simulink model "spacecraft_animation"  (Simulink 9.2)
settings: Solver=ode45  StartTime=0.0  StopTime=10000  RelTol=1e-3  EnableMultiTasking=on
undefined symbols (not defined in the file or in its folder): drawSpacecraft
libraries: simulink x6
settings Model: Creator=beard  LastModifiedBy=beard
settings OptimizationCC: ExpressionDepthLimit=2147483647  InitFltsAndDblsToZero=on
settings DebuggingCC: SolverPrmCheckMsg=warning
settings GRTTargetCC: GeneratePreprocessorConditionals=Use local settings
settings ConfigComp: CovExternalEMLEnable=on

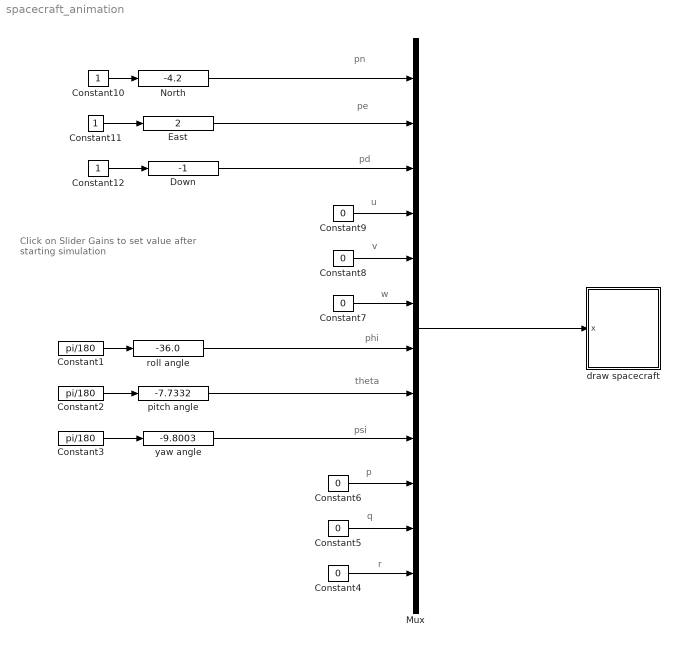
== system spacecraft_animation ==
  note: pn
  note: pe
  note: pd
  note: phi
  note: theta
  note: psi
  note: p
  note: q
  note: r
  note: u
  note: v
  note: w
  note: Click on Slider Gains to set value
      | after starting simulation
  Constant1 : Constant  Value=pi/180
  Constant10 : Constant
  Constant11 : Constant
  Constant12 : Constant
  Constant2 : Constant  Value=pi/180
  Constant3 : Constant  Value=pi/180
  Constant{4..9} (6 alike) : Constant  Value=0
  Down : simulink/Math Operations/Slider Gain  gain=-1  low=-10  high=10
  East : simulink/Math Operations/Slider Gain  gain=2  low=-10  high=10
  Mux : Mux  Inputs=12
  North : simulink/Math Operations/Slider Gain  gain=-4.2  low=-10  high=10
  draw spacecraft : Subsystem
      mask init:
      | % Define the vertices (physical location of vertices
      |   V = [...
      | 	 1    1    0;... % point 1
      |      1   -1    0;... % point 2
      |     -1   -1    0;... % point 3
      |     -1    1    0;... % point 4
      | 	 1    1   -2;... % point 5
      |      1   -1   -2;... % point 6
      |     -1   -1   -2;... % point 7
      |     -1    1   -2;... % point 8
      | 	 1.5  1.5  0;... % point 9
      |      1.5 -1.5  0;... % point 10
      |     -1.5 -1.5  0;... % point 11
      |     -1.5  1.5  0;... % point 12
      |   ];
      | 
      | % define faces as a list of vertices numbered above
      |   F = [...
      |         1, 2,  6,  5;...  % front
      |         4, 3,  7,  8;...  % back
      |         1, 5,  8,  4;...  % right 
      |         2, 6,  7,  3;...  % left
      |         5, 6,  7,  8;...  % top
      |         9, 10, 11, 12;... % bottom
      |         ];
      | 
      | % define colors for each face    
      |   myred = [1, 0, 0];
      |   mygreen = [0, 1, 0];
      |   myblue = [0, 0, 1];
      |   myyellow = [1, 1, 0];
      |   mycyan = [0, 1, 1];
      | 
      |   patchcolors = [...
      |     myred;...    % front
      |     mygreen;...  % back
      |     myblue;...   % right
      |     myyellow;... % left
      |     mycyan;...   % top
      |     mycyan;...   % bottom
      |     ];
      mask Display: image(imread('tv.jpg'))
  pitch angle : simulink/Math Operations/Slider Gain  gain=-7.7332  low=-180  high=180
  roll angle : simulink/Math Operations/Slider Gain  gain=-36.0  low=-180  high=180
  "yaw angle " : simulink/Math Operations/Slider Gain  gain=-9.8003  low=-180  high=180
  wires:
  Mux/1 -> draw spacecraft/1(x)
  roll angle/1 -> Mux/7
  Constant1/1 -> roll angle/1
  pitch angle/1 -> Mux/8
  Constant2/1 -> pitch angle/1
  "yaw angle "/1 -> Mux/9
  Constant3/1 -> "yaw angle "/1
  Constant4/1 -> Mux/12
  Constant5/1 -> Mux/11
  Constant6/1 -> Mux/10
  Constant7/1 -> Mux/6
  Constant8/1 -> Mux/5
  Constant9/1 -> Mux/4
  North/1 -> Mux/1
  Constant10/1 -> North/1
  East/1 -> Mux/2
  Constant11/1 -> East/1
  Down/1 -> Mux/3
  Constant12/1 -> Down/1

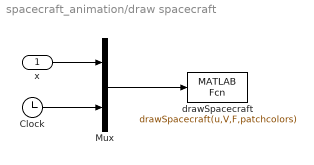
== system spacecraft_animation/draw spacecraft ==
  x : Inport
  Clock : Clock
  Mux : Mux  Inputs=2
  drawSpacecraft : MATLABFcn  MATLABFcn=drawSpacecraft(u,V,F,patchcolors)  OutputDimensions=0  SampleTime=0.1
  wires:
  Mux/1 -> drawSpacecraft/1
  x/1 -> Mux/1
  Clock/1 -> Mux/2
